simulink model "PDCj31"  (R2016b)
settings: Solver=VariableStepAuto  StartTime=0.0  StopTime=100  RelTol=1e-3
values from neighbouring files (symbols this model uses):
  A = [-0.003401570000000  -0.000000016230000 ... (first row only)    [Lyglobal.m]
  A1 = [-0.002786000000000  -0.000000019880000 ... (first row only)    [Lyglobal.m]
  B = [1;0]    [Lyglobal.m]
  B1 = [1;0]    [Lyglobal.m]
  C = [1 0]    [Lyglobal.m]
  C1 = [1 0]    [Lyglobal.m]
  D = 0    [Lyglobal.m]
  D1 = 0    [Lyglobal.m]
  K = [8.997598430000000   0.008999983770000]    [Lyglobal.m]    (also in PDCtracking.m = [K k]; planta.m = acker(A,B,P))
  K1 = [7.997223999999999   0.000079980120000]    [Lyglobal.m]    (also in Planta100.m = acker(A1,B1,P))
libraries: fuzblock x4
settings Model: Creator=Dell  LastModifiedBy=Dell

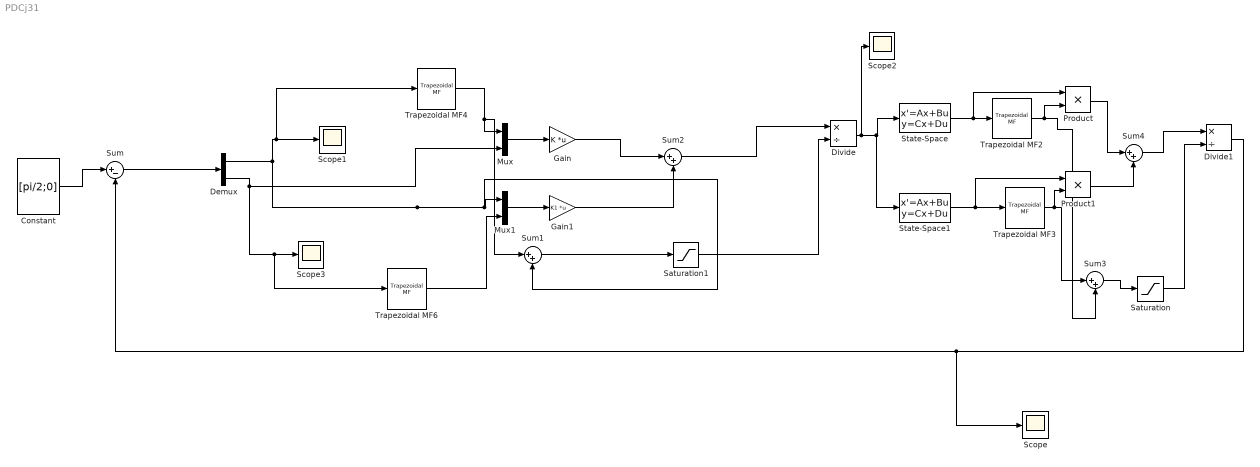
== system PDCj31 ==
  Constant : Constant  Value=[pi/2;0]  VectorParams1D=off
  Demux : Demux  Outputs=2
  Divide : Product  Inputs=*/
  Divide1 : Product  Inputs=*/
  Gain : Gain  Gain=K  Multiplication=Matrix(K*u)
  Gain1 : Gain  Gain=K1  Multiplication=Matrix(K*u)
  Mux : Mux  Inputs=2
  Mux1 : Mux  Inputs=2
  Product : Product
  Product1 : Product
  Saturation : Saturate  UpperLimit=1  LowerLimit=0.0001
  Saturation1 : Saturate  UpperLimit=1  LowerLimit=.0001
  Scope{,1..3} (4 alike) : Scope
  State-Space : StateSpace  A=A  B=B  C=C  D=D  X0=0
  State-Space1 : StateSpace  A=A1  B=B1  C=C1  D=D1  X0=0
  Sum : Sum  Inputs=|+-
  Sum{1..4} (4 alike) : Sum  Inputs=|++
  Trapezoidal MF2 : fuzblock/Membership  Functions/Trapezoidal MF  a=-1  b=50  c=75  d=100
  Trapezoidal MF3 : fuzblock/Membership  Functions/Trapezoidal MF  a=1  b=-50  c=-75  d=-100
  Trapezoidal MF4 : fuzblock/Membership  Functions/Trapezoidal MF  a=-1  b=50  c=75  d=100
  Trapezoidal MF6 : fuzblock/Membership  Functions/Trapezoidal MF  a=-1  b=-25  c=-50  d=-100
  wires:
  Constant/1 -> Sum/1
  Mux/1 -> Gain/1
  Sum2/1 -> Divide/1
  Gain/1 -> Sum2/1
  Gain1/1 -> Sum2/2
  Divide/1 -> Scope2/1, State-Space1/1, State-Space/1
  State-Space/1 -> Product/1, Trapezoidal MF2/1
  State-Space1/1 -> Product1/1, Trapezoidal MF3/1
  Trapezoidal MF3/1 -> Product1/2, Sum3/1
  Trapezoidal MF2/1 -> Product/2, Sum3/2
  Divide1/1 -> Scope/1, Sum/2
  Sum3/1 -> Saturation/1
  Saturation/1 -> Divide1/2
  Sum1/1 -> Saturation1/1
  Saturation1/1 -> Divide/2
  Sum/1 -> Demux/1
  Trapezoidal MF4/1 -> Sum1/1, Mux/1
  Demux/1 -> Trapezoidal MF4/1, Scope1/1, Sum1/2, Mux1/1
  Mux1/1 -> Gain1/1
  Demux/2 -> Mux/2, Trapezoidal MF6/1, Scope3/1
  Trapezoidal MF6/1 -> Mux1/2
  Product1/1 -> Sum4/2
  Product/1 -> Sum4/1
  Sum4/1 -> Divide1/1
